simulink model "bandwidth_model"  (R2024a)
settings: Solver=VariableStepAuto  StartTime=0.0  StopTime=Inf  RelTol=1e-3
values from neighbouring files (symbols this model uses):
  GV_den = [1 1021 4845]    [lecture_bandwidth.m]
  GV_num = [46163]    [lecture_bandwidth.m]
libraries: aerolibanimutils x1
settings Model: Creator=Christopher  LastModifiedBy=chris
settings SolverCC: AlgebraicLoopSolver=TrustRegion
settings DataIOCC: ReturnWorkspaceOutputs=off
settings DebuggingCC: UnconnectedInputMsg=warning  UnconnectedOutputMsg=warning  UnconnectedLineMsg=warning  ArithmeticOperatorsInVariantConditions=warning
settings ModelReferenceCC: EnableRefExpFcnMdlSchedulingChecks=on
settings SFSimCC: CustomCodeUndefinedFunction=UseInterfaceOnly
settings RTWCC: GPUComputeCapability=3.5

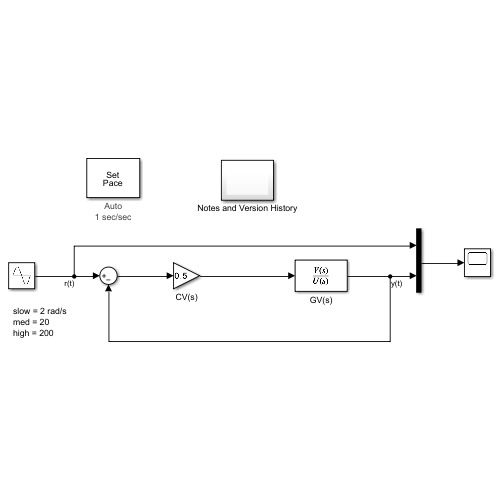
[thumbnail: Simulink's stored preview of the top-level diagram]
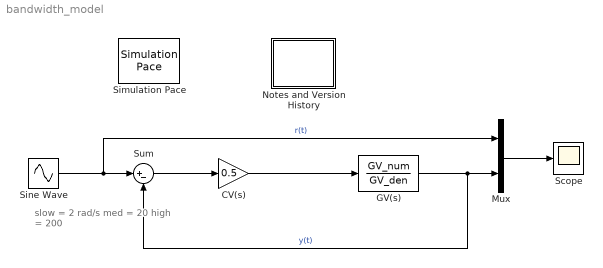
== system bandwidth_model ==
  note: slow = 2 rad/s
      | med = 20
      | high = 200
  CV(s) : Gain  Gain=0.5
  GV(s) : TransferFcn  Numerator=GV_num  Denominator=GV_den
  Mux : Mux  Inputs=2
  Notes and Version History : Subsystem
  Scope : Scope
  Simulation Pace : aerolibanimutils/Simulation Pace  SimulationPace=1  SleepMode=Auto  OutputPaceError=off  SampleTime=1/30
  Sine Wave : Sin  Frequency=50  SampleTime=0
  Sum : Sum  Inputs=|+-
  wires:
  GV(s)/1 -> Mux/2, Sum/2  "y(t)"
  Sum/1 -> CV(s)/1
  Sine Wave/1 -> Mux/1, Sum/1  "r(t)"
  CV(s)/1 -> GV(s)/1
  Mux/1 -> Scope/1

== system bandwidth_model/Notes and Version History ==
  note: Verify bandwidth calculations
      |
      | Christopher Lum
      | lum@uw.edu
      |
      | Version History
      | 05/10/19: Created
      | 01/07/25: Updated documentation
